simulink model "M2C_IM_CL_V1_NCADMM_Sim"  (R2023a)
settings: Solver=ode4  StartTime=0.0  StopTime=t_sim  FixedStep=tsim  RelTol=1e-3
model workspace (MAT data in the model file):
  global_can_baud_rate = '1000000'
  global_ip_addresses : object (value not decoded)
values from neighbouring files (symbols this model uses):
  A = [1 1 1 0 0 0 ... (first row only)    [M2C_init.m]    (also in MMCC_Sim_Script_BCD_activeset.m = -[1 0 0 1 0 0 1 0 0; 0 1 0 0 1 0 0 1 0; 0 0 1 0 0 1 0 0 1; -; MMCC_Sim_Script_BCD_activeset_LH.m = -[1 0 0 1 0 0 1 0 0; 0 1 0 0 1 0 0 1 0; 0 0 1 0 0 1 0 0 1; -)
  A11 = -(1/tau_sig)*eye(2)    [M2C_init.m]
  A21 = (Lm/tau_r)*eye(2)    [M2C_init.m]
  A_admm = zeros(2*Np, Np)    [M2C_init.m]
  A_cc = [1 0 ... (first row only)    [M2C_init.m]
  b_admm_1 = imax_admm*ones(2*Np,1)    [M2C_init.m]
  b_cc = Vmax_cc*ones(4,1)    [M2C_init.m]
  c_admm = -imax_admm*ones(Np,1)    [M2C_init.m]
  C_obs = [eye(2) zeros(2)]    [M2C_init.m]
  C_sm = 987e-6    (= 0.000987)    [M2C_init.m]
  G_cc = [1 1 ... (first row only)    [M2C_init.m]
  J_imag = [0 -1 ... (first row only)    [M2C_init.m]
  K_obsm = K_obs2'    [M2C_init.m]
  K_obsp = K_obs1'    [M2C_init.m]
  kr = Lm/Lr    (= 0.989061842659)    [M2C_init.m]
  L = 5e-3    (= 0.005)    [M2C_init.m]    (also in MMCC_Sim_Script_BCD_activeset.m = 0.02; MMCC_Sim_Script_BCD_activeset_LH.m = 0.02)
  Lsigmar = 2.6e-3    (= 0.0026)    [M2C_init.m]
  Lsigmas = 2.6e-3    (= 0.0026)    [M2C_init.m]
  N = [1/sqrt(3) 0;-1/(2*sqrt(3)) 1/2;-1/(2*sqrt(3)) -1/2;-1/sqrt(3) 0;1/(2*sqrt(3)) -1/2;1/(2*sqrt(3)) 1/2]    [M2C_init.m]    (also in MMCC_Sim_Script_BCD_activeset.m = null(A,'rational'); MMCC_Sim_Script_BCD_activeset_LH.m = [-0.4430   -0.4780    0.0994    0.0994)
  n = 4    [M2C_init.m]
  p = 2    [M2C_init.m]
  phirN = 1*Vb/ws_nom    [M2C_init.m]
  prmt_ADMM = [n, lambda_z, rho, lambda_e, C_sm, Np, imax_admm]    [M2C_init.m]
  prmt_bkpsi = [ts, Np, lambda_o, imax_admm]    [M2C_init.m]
  prmt_CCMPC = [ts, L, lambda_u, lambda_i, R, e]    [M2C_init.m]
  prmt_OBS = [ts, kr, sigma, Ls, tau_r]    [M2C_init.m]
  R = 0.2    [M2C_init.m]    (also in MMCC_Sim_Script_BCD_activeset.m = 0.001; MMCC_Sim_Script_BCD_activeset_LH.m = 0.001)
  Rr = 1.8    [M2C_init.m]
  Rs = 1.8    [M2C_init.m]
  Rsig = Rs + Rr*kr^2    (= 3.56083799149)    [M2C_init.m]
  SN = PN/FPn    (= 3703.7037037)    [M2C_init.m]
  T = [An ... (first row only)    [M2C_init.m]    (also in MMCC_Sim_Script_BCD_activeset.m = [1   0 ; -1/2  sqrt(3)/2; -1/2  -sqrt(3)/2]; MMCC_Sim_Script_BCD_activeset_LH.m = [1   0 ; -1/2  sqrt(3)/2; -1/2  -sqrt(3)/2])
  t_arranque = t_flux + 5/(dam*wn_flux) + 0.4    [M2C_init.m]
  t_flux = t_maq + 0.1    (= 0.3)    [M2C_init.m]
  t_load = t_arranque    [M2C_init.m]
  Tab0 = (1/3)*[2 -1 -1 ... (first row only)    [M2C_init.m]
  Tabc = [1 0; -.5 sqrt(3)/2; -.5 -sqrt(3)/2]    [M2C_init.m]
  tau_r = Lr/Rr    (= 0.132055555556)    [M2C_init.m]
  TN = PN/(nN*pi/30)    (= 19.7571653493)    [M2C_init.m]
  ts = 1/fs    (= 0.000166666666667)    [M2C_init.m]
  tsim = ts/40    (= 4.16666666667e-06)    [M2C_init.m]
  Vc0 = n*Vc_sm    (= 520)    [M2C_init.m]    (also in MMCC_Sim_Script_BCD_activeset.m = 18000; MMCC_Sim_Script_BCD_activeset_LH.m = 18000)
  Vc_sm = 130    [M2C_init.m]
  Vdc = n*Vc_sm    (= 520)    [M2C_init.m]
undefined symbols (not defined in the file or in its folder): Down, M2C_ADMM_Init_IM_V1, plecs, Up
libraries: spsIGBTDiodeLib x48, spsVoltageMeasurementLib x36, spsSeriesRLCBranchLib x30, spsCurrentMeasurementLib x10, eePwmGenerator x6, rtlab x3, dspstat3 x2, spsControlledVoltageSourceLib x2, spsDCVoltageSourceLib x2, opal_lib x1, dspfdesign x1, spsMeanLib x1
(part 4 of 6)

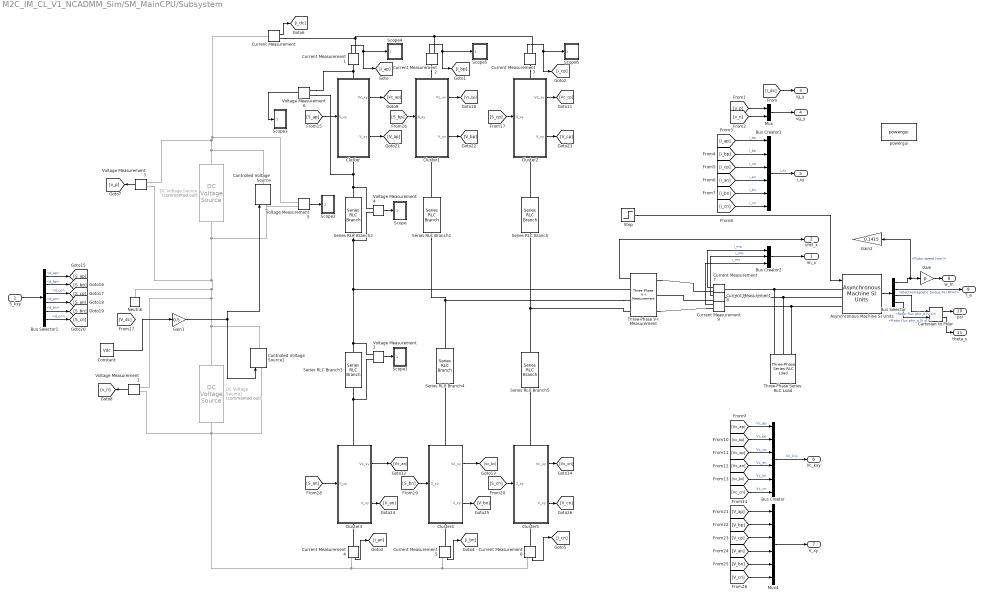
== system M2C_IM_CL_V1_NCADMM_Sim/SM_MainCPU/Subsystem ==
  S_kxy : Inport
  Asynchronous Machine SI Units : spsAsynchronousMachineSIUnitsLib/Asynchronous Machine SI Units  RotorType=Squirrel-cage  PresetModel=No  MechanicalLoad=Torque Tm  ShowDetailedParameters=on  ReferenceFrame=Rotor  Units=SI  MeasurementBus=off  NominalParameters=[3000 400 50]  VoltageRatio=1  Stator=[Rs Lsigmas]  Rotor=[Rr Lsigmar]  Cage1=[0.4155 0.002066]  Cage2=[0.4168 0.0003495]  Lm=Lm  Mechanical=[0.006 0.0057*0 p]  PolePairs=2  InitialConditions=[1 90 0 0 0 0 0 0]  SimulateSaturation=off  Saturation=[14.03593122, 27.81365428, 53.79336849, 72.68890987, 97.98006896, 148.6815601, 215.7428561, 302.9841135, 428.7778367 ; 230, 322, 414, 460, 506, 552, 598, 644, 690]  LoadFlowParameters=1492000  TsPowergui=0  TsBlock=tsim  IterativeModel=Trapezoidal non iterative  IterativeDiscreteModel=Trapezoidal non iterative  Pmec=0
  Bus Creator : BusCreator  Inputs=6
  Bus Creator1 : BusCreator  Inputs=6
  Bus Creator2 : BusCreator  Inputs=3
  Bus Selector : BusSelector  OutputSignals=Mechanical.Rotor speed (wm),Mechanical.Electromagnetic torque Te (N*m),Rotor measurements.Rotor flux phir_d (V s),Rotor measurements.Rotor flux phir_q (V s)
  Bus Selector1 : BusSelector  OutputSignals=S_p.d_ap,S_p.d_bp,S_p.d_cp,S_n.d_an,S_n.d_bn,S_n.d_cn
  Cartesian to Polar : simulink_extras/Transformations/Cartesian to Polar
  Cluster : Subsystem
      settings: PortSchema="{\"entries\":[{\"content\":{\"sides\":[{\"content\":{\"connectorIds\":[\"In1\"]},\"type\":\"ConnectorPlacement.EquallySpacedRectSide\",\"uuid\":\"19b6a211-5636-4e1a-b566-92ce17a08f23\"},{\"content\":{\"connectorIds\":[\"Out1\",\"Out2\"],\"side\":\"RIGHT\"},\"type\":\"ConnectorPlacement.EquallySpacedRectSide\",\"uuid\":\"483b1e0d-23ae-4dba-a621-2706d89ef2c0\"},{\"content\":{\"connectorIds\":[\"LConn1\"],\"side\":\"TOP\"},\"type\":\"ConnectorPlacement.EquallySpacedRectSide\",\"uuid\":\"4d4f4f94-f98d-4d38-ba04-9db58fc318a2\"},{\"content\":{\"connectorIds\":[\"RConn1\"],\"side\":\"BOTTOM\"},\"type\":\"ConnectorPlacement.EquallySpacedRectSide\",\"uuid\":\"4e2c39e0-8a4f-4729-a37c-1f4684d26f15\"}]},\"type\":\"ConnectorPlacement.EquallySpacedConnector\",\"uuid\":\"4c9a22d5-cdf0-40e5-b6bd-94d006c5c37f\"}],\"packageUris\":[\"http://schema.mathworks.com/mf0/Connector/R2020b\"],\"version\":\"1.0\"}"
  Cluster1 : Subsystem
      settings: PortSchema="{\"entries\":[{\"content\":{\"sides\":[{\"content\":{\"connectorIds\":[\"In1\"]},\"type\":\"ConnectorPlacement.EquallySpacedRectSide\",\"uuid\":\"19b6a211-5636-4e1a-b566-92ce17a08f23\"},{\"content\":{\"connectorIds\":[\"Out1\",\"Out2\"],\"side\":\"RIGHT\"},\"type\":\"ConnectorPlacement.EquallySpacedRectSide\",\"uuid\":\"483b1e0d-23ae-4dba-a621-2706d89ef2c0\"},{\"content\":{\"connectorIds\":[\"LConn1\"],\"side\":\"TOP\"},\"type\":\"ConnectorPlacement.EquallySpacedRectSide\",\"uuid\":\"4d4f4f94-f98d-4d38-ba04-9db58fc318a2\"},{\"content\":{\"connectorIds\":[\"RConn1\"],\"side\":\"BOTTOM\"},\"type\":\"ConnectorPlacement.EquallySpacedRectSide\",\"uuid\":\"4e2c39e0-8a4f-4729-a37c-1f4684d26f15\"}]},\"type\":\"ConnectorPlacement.EquallySpacedConnector\",\"uuid\":\"4c9a22d5-cdf0-40e5-b6bd-94d006c5c37f\"}],\"packageUris\":[\"http://schema.mathworks.com/mf0/Connector/R2020b\"],\"version\":\"1.0\"}"
  Cluster2 : Subsystem
      settings: PortSchema="{\"entries\":[{\"content\":{\"sides\":[{\"content\":{\"connectorIds\":[\"In1\"]},\"type\":\"ConnectorPlacement.EquallySpacedRectSide\",\"uuid\":\"19b6a211-5636-4e1a-b566-92ce17a08f23\"},{\"content\":{\"connectorIds\":[\"Out1\",\"Out2\"],\"side\":\"RIGHT\"},\"type\":\"ConnectorPlacement.EquallySpacedRectSide\",\"uuid\":\"483b1e0d-23ae-4dba-a621-2706d89ef2c0\"},{\"content\":{\"connectorIds\":[\"LConn1\"],\"side\":\"TOP\"},\"type\":\"ConnectorPlacement.EquallySpacedRectSide\",\"uuid\":\"4d4f4f94-f98d-4d38-ba04-9db58fc318a2\"},{\"content\":{\"connectorIds\":[\"RConn1\"],\"side\":\"BOTTOM\"},\"type\":\"ConnectorPlacement.EquallySpacedRectSide\",\"uuid\":\"4e2c39e0-8a4f-4729-a37c-1f4684d26f15\"}]},\"type\":\"ConnectorPlacement.EquallySpacedConnector\",\"uuid\":\"4c9a22d5-cdf0-40e5-b6bd-94d006c5c37f\"}],\"packageUris\":[\"http://schema.mathworks.com/mf0/Connector/R2020b\"],\"version\":\"1.0\"}"
  Cluster3 : Subsystem
      settings: PortSchema="{\"entries\":[{\"content\":{\"sides\":[{\"content\":{\"connectorIds\":[\"In1\"]},\"type\":\"ConnectorPlacement.EquallySpacedRectSide\",\"uuid\":\"19b6a211-5636-4e1a-b566-92ce17a08f23\"},{\"content\":{\"connectorIds\":[\"Out1\",\"Out2\"],\"side\":\"RIGHT\"},\"type\":\"ConnectorPlacement.EquallySpacedRectSide\",\"uuid\":\"483b1e0d-23ae-4dba-a621-2706d89ef2c0\"},{\"content\":{\"connectorIds\":[\"LConn1\"],\"side\":\"TOP\"},\"type\":\"ConnectorPlacement.EquallySpacedRectSide\",\"uuid\":\"4d4f4f94-f98d-4d38-ba04-9db58fc318a2\"},{\"content\":{\"connectorIds\":[\"RConn1\"],\"side\":\"BOTTOM\"},\"type\":\"ConnectorPlacement.EquallySpacedRectSide\",\"uuid\":\"4e2c39e0-8a4f-4729-a37c-1f4684d26f15\"}]},\"type\":\"ConnectorPlacement.EquallySpacedConnector\",\"uuid\":\"4c9a22d5-cdf0-40e5-b6bd-94d006c5c37f\"}],\"packageUris\":[\"http://schema.mathworks.com/mf0/Connector/R2020b\"],\"version\":\"1.0\"}"
  Cluster4 : Subsystem
      settings: PortSchema="{\"entries\":[{\"content\":{\"sides\":[{\"content\":{\"connectorIds\":[\"In1\"]},\"type\":\"ConnectorPlacement.EquallySpacedRectSide\",\"uuid\":\"19b6a211-5636-4e1a-b566-92ce17a08f23\"},{\"content\":{\"connectorIds\":[\"Out1\",\"Out2\"],\"side\":\"RIGHT\"},\"type\":\"ConnectorPlacement.EquallySpacedRectSide\",\"uuid\":\"483b1e0d-23ae-4dba-a621-2706d89ef2c0\"},{\"content\":{\"connectorIds\":[\"LConn1\"],\"side\":\"TOP\"},\"type\":\"ConnectorPlacement.EquallySpacedRectSide\",\"uuid\":\"4d4f4f94-f98d-4d38-ba04-9db58fc318a2\"},{\"content\":{\"connectorIds\":[\"RConn1\"],\"side\":\"BOTTOM\"},\"type\":\"ConnectorPlacement.EquallySpacedRectSide\",\"uuid\":\"4e2c39e0-8a4f-4729-a37c-1f4684d26f15\"}]},\"type\":\"ConnectorPlacement.EquallySpacedConnector\",\"uuid\":\"4c9a22d5-cdf0-40e5-b6bd-94d006c5c37f\"}],\"packageUris\":[\"http://schema.mathworks.com/mf0/Connector/R2020b\"],\"version\":\"1.0\"}"
  Cluster5 : Subsystem
      settings: PortSchema="{\"entries\":[{\"content\":{\"sides\":[{\"content\":{\"connectorIds\":[\"In1\"]},\"type\":\"ConnectorPlacement.EquallySpacedRectSide\",\"uuid\":\"19b6a211-5636-4e1a-b566-92ce17a08f23\"},{\"content\":{\"connectorIds\":[\"Out1\",\"Out2\"],\"side\":\"RIGHT\"},\"type\":\"ConnectorPlacement.EquallySpacedRectSide\",\"uuid\":\"483b1e0d-23ae-4dba-a621-2706d89ef2c0\"},{\"content\":{\"connectorIds\":[\"LConn1\"],\"side\":\"TOP\"},\"type\":\"ConnectorPlacement.EquallySpacedRectSide\",\"uuid\":\"4d4f4f94-f98d-4d38-ba04-9db58fc318a2\"},{\"content\":{\"connectorIds\":[\"RConn1\"],\"side\":\"BOTTOM\"},\"type\":\"ConnectorPlacement.EquallySpacedRectSide\",\"uuid\":\"4e2c39e0-8a4f-4729-a37c-1f4684d26f15\"}]},\"type\":\"ConnectorPlacement.EquallySpacedConnector\",\"uuid\":\"4c9a22d5-cdf0-40e5-b6bd-94d006c5c37f\"}],\"packageUris\":[\"http://schema.mathworks.com/mf0/Connector/R2020b\"],\"version\":\"1.0\"}"
  Constant : Constant  Value=Vdc  SampleTime=ts
  Controlled Voltage Source : spsControlledVoltageSourceLib/Controlled Voltage Source  Initialize=on  Source_Type=AC  Amplitude=0  Phase=0  Frequency=0  Measurements=None
  Controlled Voltage Source1 : spsControlledVoltageSourceLib/Controlled Voltage Source  Initialize=on  Source_Type=AC  Amplitude=0  Phase=0  Frequency=0  Measurements=None
  Current Measurement{,1..9} (10 alike) : spsCurrentMeasurementLib/Current Measurement  PhasorSimulation=off  OutputType=Complex  PSBequivalent=0
  DC Voltage Source : spsDCVoltageSourceLib/DC Voltage Source  Commented=on  Amplitude=Vdc/2  Measurements=None
  DC Voltage Source1 : spsDCVoltageSourceLib/DC Voltage Source  Commented=on  Amplitude=Vdc/2  Measurements=None
  Gain : Gain  Gain=p
  Gain1 : Gain  Gain=0.5
  Gain2 : Gain  Gain=0.1415
  Mux : Mux  Inputs=2
  Mux4 : Mux  Inputs=6
  Neutral : spsNeutralLib/Neutral  LConnTagsString=a  NodeNumber=10
      settings: AttributesFormatString=node %<NodeNumber>
  Scope : Subsystem  LoadFcn=plecs('sl', 300);  InitFcn=plecs('sl', 314);  StartFcn=plecs('sl', 308);  StopFcn=plecs('sl', 309);  mask{Settings=<binary blob, 1052 chars, not shown>}
      mask init:
      | plecs('sl', 315);
      settings: CopyFcn=plecs('sl', 303);  DeleteFcn=plecs('sl', 305);  UndoDeleteFcn=plecs('sl', 306);  PreSaveFcn=plecs('sl', 311);  NameChangeFcn=plecs('sl', 310);  DestroyFcn=plecs('sl', 307);  OpenFcn=plecs('sl', 302);  ErrorFcn=plerrorfcn
      mask Display: plot([0.1 0.9 0.9 0.1 0.1], [0.9 0.9 0.5 0.5 0.9])
  Scope1 : Subsystem  LoadFcn=plecs('sl', 300);  InitFcn=plecs('sl', 314);  StartFcn=plecs('sl', 308);  StopFcn=plecs('sl', 309);  mask{Settings=<binary blob, 1052 chars, not shown>}
      mask init:
      | plecs('sl', 315);
      settings: CopyFcn=plecs('sl', 303);  DeleteFcn=plecs('sl', 305);  UndoDeleteFcn=plecs('sl', 306);  PreSaveFcn=plecs('sl', 311);  NameChangeFcn=plecs('sl', 310);  DestroyFcn=plecs('sl', 307);  OpenFcn=plecs('sl', 302);  ErrorFcn=plerrorfcn
      mask Display: plot([0.1 0.9 0.9 0.1 0.1], [0.9 0.9 0.5 0.5 0.9])
  Scope2 : Subsystem  LoadFcn=plecs('sl', 300);  InitFcn=plecs('sl', 314);  StartFcn=plecs('sl', 308);  StopFcn=plecs('sl', 309);  mask{Settings=<binary blob, 1052 chars, not shown>}
      mask init:
      | plecs('sl', 315);
      settings: CopyFcn=plecs('sl', 303);  DeleteFcn=plecs('sl', 305);  UndoDeleteFcn=plecs('sl', 306);  PreSaveFcn=plecs('sl', 311);  NameChangeFcn=plecs('sl', 310);  DestroyFcn=plecs('sl', 307);  OpenFcn=plecs('sl', 302);  ErrorFcn=plerrorfcn
      mask Display: plot([0.1 0.9 0.9 0.1 0.1], [0.9 0.9 0.5 0.5 0.9])
  Scope3 : Subsystem  LoadFcn=plecs('sl', 300);  InitFcn=plecs('sl', 314);  StartFcn=plecs('sl', 308);  StopFcn=plecs('sl', 309);  mask{Settings=<binary blob, 1052 chars, not shown>}
      mask init:
      | plecs('sl', 315);
      settings: CopyFcn=plecs('sl', 303);  DeleteFcn=plecs('sl', 305);  UndoDeleteFcn=plecs('sl', 306);  PreSaveFcn=plecs('sl', 311);  NameChangeFcn=plecs('sl', 310);  DestroyFcn=plecs('sl', 307);  OpenFcn=plecs('sl', 302);  ErrorFcn=plerrorfcn
      mask Display: plot([0.1 0.9 0.9 0.1 0.1], [0.9 0.9 0.5 0.5 0.9])
  Scope4 : Subsystem  LoadFcn=plecs('sl', 300);  InitFcn=plecs('sl', 314);  StartFcn=plecs('sl', 308);  StopFcn=plecs('sl', 309);  mask{Settings=<binary blob, 236 chars, not shown>}
      mask init:
      | plecs('sl', 315);
      settings: CopyFcn=plecs('sl', 303);  DeleteFcn=plecs('sl', 305);  UndoDeleteFcn=plecs('sl', 306);  PreSaveFcn=plecs('sl', 311);  NameChangeFcn=plecs('sl', 310);  DestroyFcn=plecs('sl', 307);  OpenFcn=plecs('sl', 302);  ErrorFcn=plerrorfcn
      mask Display: plot([0.1 0.9 0.9 0.1 0.1], [0.9 0.9 0.5 0.5 0.9])
  Scope5 : Subsystem  LoadFcn=plecs('sl', 300);  InitFcn=plecs('sl', 314);  StartFcn=plecs('sl', 308);  StopFcn=plecs('sl', 309);  mask{Settings=<binary blob, 236 chars, not shown>}
      mask init:
      | plecs('sl', 315);
      settings: CopyFcn=plecs('sl', 303);  DeleteFcn=plecs('sl', 305);  UndoDeleteFcn=plecs('sl', 306);  PreSaveFcn=plecs('sl', 311);  NameChangeFcn=plecs('sl', 310);  DestroyFcn=plecs('sl', 307);  OpenFcn=plecs('sl', 302);  ErrorFcn=plerrorfcn
      mask Display: plot([0.1 0.9 0.9 0.1 0.1], [0.9 0.9 0.5 0.5 0.9])
  Scope6 : Subsystem  LoadFcn=plecs('sl', 300);  InitFcn=plecs('sl', 314);  StartFcn=plecs('sl', 308);  StopFcn=plecs('sl', 309);  mask{Settings=<binary blob, 236 chars, not shown>}
      mask init:
      | plecs('sl', 315);
      settings: CopyFcn=plecs('sl', 303);  DeleteFcn=plecs('sl', 305);  UndoDeleteFcn=plecs('sl', 306);  PreSaveFcn=plecs('sl', 311);  NameChangeFcn=plecs('sl', 310);  DestroyFcn=plecs('sl', 307);  OpenFcn=plecs('sl', 302);  ErrorFcn=plerrorfcn
      mask Display: plot([0.1 0.9 0.9 0.1 0.1], [0.9 0.9 0.5 0.5 0.9])
  Series RLC Branch{,1..5} (6 alike) : spsSeriesRLCBranchLib/Series RLC Branch  LConnTagsString=__new0  RConnTagsString=__new0  BranchType=RL  Resistance=R  Inductance=L  SetiL0=off  InitialCurrent=0  Capacitance=1e-6  Setx0=off  InitialVoltage=0  Measurements=None
  Step : Step  Time=t_load+2  After=TN*0.4  SampleTime=0
  Three-Phase Series RLC Load : spsThreePhaseSeriesRLCLoadLib/Three-Phase Series RLC Load  LConnTagsString=A|B|C  Configuration=Y (floating)  NominalVoltage=VLLN  Vabc=[1e3 1e3 1e3]  Vabcp=[1e3 1e3 1e3]  NominalFrequency=50  UnbalancedPower=off  ActivePower=SN*0.01  InductivePower=0  CapacitivePower=0  Pabc=[10e3 9e3 11e3]  QLabc=[100 90 110]  QCabc=[100 90 110]  Pabcp=[10e3 9e3 11e3]  QLabcp=[100 90 110]  QCabcp=[100 90 110]  Measurements=None  LoadType=constant Z
  Three-Phase V-I Measurement : spsThreePhaseVIMeasurementLib/Three-Phase V-I Measurement  VoltageMeasurement=phase-to-phase  SetLabelV=off  LabelV=Vabc  Vpu=off  VpuLL=off  CurrentMeasurement=no  SetLabelI=off  LabelI=Iabc  Ipu=off  Pbase=100e6  Vbase=500e3  OutputType=Complex  PhasorSimulation=off  PSBequivalent=0
  Voltage Measurement{1..6} (6 alike) : spsVoltageMeasurementLib/Voltage Measurement  PhasorSimulation=off  OutputType=Complex  PSBequivalent=0
  powergui : spspowerguiLib/powergui  Priority=1  SimulationMode=Discrete  SampleTime=tsim  frequency=60  Iterations=50  frequencyindice=0  Pbase=100e6  ErrMax=1e-4  UnitsV=kV  UnitsW=MW  buscounter=0  FunctionMessages=off  echomessages=off  EnableUseOfTLC=off  CurrentSourceSwitches=off  DisableSnubberDevices=off  DisableRonSwitches=off  DisableVfSwitches=off  DisplayEquations=off  AutomaticDiscreteSolvers=off  SolverType=Tustin/Backward Euler (TBE)  Interpol=off  ExternalGateDelay=off  methode=off  Ts=100  x0status=blocks  SPID=on  SwTol=0  HookPort=off  NonlinearTolerance=1e-4  nMaxIteration=100  ContinueOnMaxIteration=off  RestoreLinks=warning  ResistiveCurrentMeasurement=off  Frange=[0:2:500]  Ylog=off  Xlog=on  ShowGrid=off  save=off  variable=ZData  structure=0  ZoomFFT=off  StartTime=0.0  cycles=1  DisplayStyle=1  fundamental=60  FreqAxis=off  MaxFrequency=1000  frequencyindicesteady=1  RmsSteady=1  display=off
  im_x : Outport
  vmll_x : Outport  Port=2
  ig_y : Outport  Port=3
  vg_y : Outport  Port=4
  i_xy : Outport  Port=5
  Vc_kxy : Outport  Port=6
  V_xy : Outport  Port=7
  w_m : Outport  Port=8
  T_e : Outport  Port=9
  psi : Outport  Port=10
  theta_s : Outport  Port=11
  wires:
  Three-Phase V-I Measurement/1 -> vmll_x/1
  [i_dc] -> ig_y/1
  Voltage Measurement3/1 -> [v_p]
  Voltage Measurement1/1 -> [v_n]
  [v_p] -> Mux/1
  [v_n] -> Mux/2
  Mux/1 -> vg_y/1
  [i_ap] -> Bus Creator1/1  "i_ap"
  [i_bp] -> Bus Creator1/2  "i_bp"
  [i_cp] -> Bus Creator1/3  "i_cp"
  [i_an] -> Bus Creator1/4  "i_an"
  [i_bn] -> Bus Creator1/5  "i_bn"
  [i_cn] -> Bus Creator1/6  "i_cn"
  Bus Creator1/1 -> i_xy/1  "i_xy"
  Cluster/1(Vc_xy) -> [Vc_ap]
  Cluster1/1(Vc_xy) -> [Vc_bp]
  Cluster2/1(Vc_xy) -> [Vc_cp]
  Cluster3/1(Vc_xy) -> [Vc_an]
  Cluster4/1(Vc_xy) -> [Vc_bn]
  Cluster5/1(Vc_xy) -> [Vc_cn]
  [Vc_ap] -> Bus Creator/1  "Vc_ap"
  [Vc_bp] -> Bus Creator/2  "Vc_bp"
  [Vc_cp] -> Bus Creator/3  "Vc_cp"
  [Vc_an] -> Bus Creator/4  "Vc_an"
  [Vc_cn] -> Bus Creator/6  "Vc_cn"
  [Vc_bn] -> Bus Creator/5  "Vc_bn"
  Bus Creator/1 -> Vc_kxy/1  "Vc_kxy"
  Bus Selector1/6 -> [S_cn]  "<d_cn>"
  Bus Selector1/5 -> [S_bn]  "<d_bn>"
  Bus Selector1/4 -> [S_an]  "<d_an>"
  Bus Selector1/3 -> [S_cp]  "<d_cp>"
  Bus Selector1/2 -> [S_bp]  "<d_bp>"
  Bus Selector1/1 -> [S_ap]  "<d_ap>"
  [S_ap] -> Cluster/1(S_xy)
  [S_bp] -> Cluster1/1(S_xy)
  [S_cp] -> Cluster2/1(S_xy)
  [S_an] -> Cluster3/1(S_xy)
  [S_bn] -> Cluster4/1(S_xy)
  [S_cn] -> Cluster5/1(S_xy)
  Bus Creator2/1 -> im_x/1
  Current Measurement1/1 -> Scope4/1(1), [i_ap]
  Current Measurement2/1 -> Scope5/1(1), [i_bp]
  Current Measurement3/1 -> Scope6/1(1), [i_cp]
  Current Measurement4/1 -> [i_an]
  Current Measurement5/1 -> [i_bn]
  Current Measurement6/1 -> [i_cn]
  Current Measurement/1 -> [i_dc]
  Current Measurement7/1 -> Bus Creator2/1  "i_ma"
  Current Measurement8/1 -> Bus Creator2/2  "i_mb"
  Current Measurement9/1 -> Bus Creator2/3  "i_mc"
  Cluster/2(V_xy) -> [V_ap]
  Cluster1/2(V_xy) -> [V_bp]
  Cluster2/2(V_xy) -> [V_cp]
  Cluster4/2(V_xy) -> [V_bn]
  Cluster5/2(V_xy) -> [V_cn]
  Cluster3/2(V_xy) -> [V_an]
  Mux4/1 -> V_xy/1
  [V_ap] -> Mux4/1
  [V_bp] -> Mux4/2
  [V_cp] -> Mux4/3
  [V_an] -> Mux4/4
  [V_bn] -> Mux4/5
  [V_cn] -> Mux4/6
  S_kxy/1 -> Bus Selector1/1
  Constant/1 -> Gain1/1
  Gain1/1 -> Controlled Voltage Source/1, Controlled Voltage Source1/1
  Asynchronous Machine SI Units/1 -> Bus Selector/1
  Bus Selector/1 -> Gain2/1, Gain/1  "<Rotor speed (wm)>"
  Gain/1 -> w_m/1
  Bus Selector/2 -> T_e/1  "<Electromagnetic torque Te (N*m)>"
  Cartesian to Polar/1 -> psi/1
  Cartesian to Polar/2 -> theta_s/1
  Bus Selector/3 -> Cartesian to Polar/1  "<Rotor flux phir_d (V s)>"
  Bus Selector/4 -> Cartesian to Polar/2  "<Rotor flux phir_q (V s)>"
  Step/1 -> Asynchronous Machine SI Units/1
  Voltage Measurement4/1 -> Scope/1(1)
  Voltage Measurement2/1 -> Scope1/1(1)
  Voltage Measurement5/1 -> Scope2/1(1)
  Voltage Measurement6/1 -> Scope3/1(1)
  connections:
  Series RLC Branch/LConn1 -- Cluster2/RConn1
  Series RLC Branch1/LConn1 -- Cluster1/RConn1
  Cluster/RConn1 -- Voltage Measurement6/LConn2 -- Voltage Measurement4/LConn1 -- Series RLC Branch2/LConn1
  Current Measurement1/RConn1 -- Current Measurement/RConn1 -- Current Measurement3/RConn1 -- Current Measurement2/RConn1
  DC Voltage Source1/LConn1 -- Controlled Voltage Source1/LConn1 -- Current Measurement4/RConn1 -- Current Measurement6/RConn1 -- Current Measurement5/RConn1 -- Voltage Measurement1/LConn1
  DC Voltage Source/RConn1 -- Controlled Voltage Source/RConn1 -- Voltage Measurement5/LConn1 -- Current Measurement/LConn1 -- Voltage Measurement3/LConn1
  Series RLC Branch3/LConn1 -- Voltage Measurement2/LConn1 -- Cluster3/LConn1
  Series RLC Branch4/LConn1 -- Cluster4/LConn1
  Series RLC Branch5/LConn1 -- Cluster5/LConn1
  Current Measurement1/LConn1 -- Voltage Measurement6/LConn1 -- Cluster/LConn1
  Current Measurement2/LConn1 -- Cluster1/LConn1
  Current Measurement3/LConn1 -- Cluster2/LConn1
  Current Measurement4/LConn1 -- Cluster3/RConn1
  Current Measurement5/LConn1 -- Cluster4/RConn1
  Current Measurement6/LConn1 -- Cluster5/RConn1
  Current Measurement7/RConn1 -- Three-Phase V-I Measurement/LConn1
  Current Measurement8/RConn1 -- Three-Phase V-I Measurement/LConn2
  Current Measurement9/RConn1 -- Three-Phase V-I Measurement/LConn3
  Three-Phase Series RLC Load/LConn1 -- Asynchronous Machine SI Units/LConn1 -- Current Measurement7/LConn1
  Three-Phase V-I Measurement/RConn3 -- Series RLC Branch/RConn1 -- Series RLC Branch5/RConn1
  DC Voltage Source/LConn1 -- Voltage Measurement5/LConn2 -- Controlled Voltage Source/LConn1 -- Neutral/LConn1 -- Voltage Measurement1/LConn2 -- Controlled Voltage Source1/RConn1 -- DC Voltage Source1/RConn1 -- Voltage Measurement3/LConn2
  Three-Phase V-I Measurement/RConn2 -- Series RLC Branch1/RConn1 -- Series RLC Branch4/RConn1
  Three-Phase Series RLC Load/LConn2 -- Asynchronous Machine SI Units/LConn2 -- Current Measurement8/LConn1
  Three-Phase Series RLC Load/LConn3 -- Asynchronous Machine SI Units/LConn3 -- Current Measurement9/LConn1
  Voltage Measurement4/LConn2 -- Three-Phase V-I Measurement/RConn1 -- Voltage Measurement2/LConn2 -- Series RLC Branch3/RConn1 -- Series RLC Branch2/RConn1

== system M2C_IM_CL_V1_NCADMM_Sim/SM_MainCPU/V REFS1 ==
  1 : Inport
  2 : Inport  Port=2
  3 : Inport  Port=3
  " 1 " : DataTypeConversion
  " 2 " : DataTypeConversion
  " 3 " : DataTypeConversion
  " InputMux " : Mux  Inputs=3
  " S-Function " : S-Function  FunctionName=plecs  SFunctionDeploymentMode=off  EnableBusSupport=off
  wires:
  " InputMux "/1 -> " S-Function "/1
  1/1 -> " 1 "/1
  " 1 "/1 -> " InputMux "/1
  2/1 -> " 2 "/1
  " 2 "/1 -> " InputMux "/2
  3/1 -> " 3 "/1
  " 3 "/1 -> " InputMux "/3

== system M2C_IM_CL_V1_NCADMM_Sim/SM_MainCPU/LCB1/Scope ==
  1 : Inport
  " InputMux " : Subsystem
      mask Display: disp('Mux')
  " S-Function " : S-Function  FunctionName=plecs  SFunctionDeploymentMode=off  EnableBusSupport=off
  wires:
  1/1 -> " InputMux "/1(In1)
  " InputMux "/1(Out) -> " S-Function "/1

== system M2C_IM_CL_V1_NCADMM_Sim/SM_MainCPU/LCB1/Scope1 ==
  1 : Inport
  " InputMux " : Subsystem
      mask Display: disp('Mux')
  " S-Function " : S-Function  FunctionName=plecs  SFunctionDeploymentMode=off  EnableBusSupport=off
  wires:
  1/1 -> " InputMux "/1(In1)
  " InputMux "/1(Out) -> " S-Function "/1

== system M2C_IM_CL_V1_NCADMM_Sim/SM_MainCPU/LCB1/Scope2 ==
  1 : Inport
  " InputMux " : Subsystem
      mask Display: disp('Mux')
  " S-Function " : S-Function  FunctionName=plecs  SFunctionDeploymentMode=off  EnableBusSupport=off
  wires:
  1/1 -> " InputMux "/1(In1)
  " InputMux "/1(Out) -> " S-Function "/1

== system M2C_IM_CL_V1_NCADMM_Sim/SM_MainCPU/LCB1/Scope5 ==
  1 : Inport
  " InputMux " : Subsystem
      mask Display: disp('Mux')
  " S-Function " : S-Function  FunctionName=plecs  SFunctionDeploymentMode=off  EnableBusSupport=off
  wires:
  1/1 -> " InputMux "/1(In1)
  " InputMux "/1(Out) -> " S-Function "/1

== system M2C_IM_CL_V1_NCADMM_Sim/SM_MainCPU/Scope/ InputMux  ==
  In1 : Inport
  Convert1 : DataTypeConversion
  Mux : Mux  Inputs=1
  Out : Outport
  wires:
  Convert1/1 -> Mux/1
  In1/1 -> Convert1/1
  Mux/1 -> Out/1

== system M2C_IM_CL_V1_NCADMM_Sim/SM_MainCPU/Scope1/ InputMux  ==
  In1 : Inport
  Convert1 : DataTypeConversion
  Mux : Mux  Inputs=1
  Out : Outport
  wires:
  Convert1/1 -> Mux/1
  In1/1 -> Convert1/1
  Mux/1 -> Out/1

== system M2C_IM_CL_V1_NCADMM_Sim/SM_MainCPU/Scope10/ InputMux  ==
  In1 : Inport
  Convert1 : DataTypeConversion
  Mux : Mux  Inputs=1
  Out : Outport
  wires:
  Convert1/1 -> Mux/1
  In1/1 -> Convert1/1
  Mux/1 -> Out/1

== system M2C_IM_CL_V1_NCADMM_Sim/SM_MainCPU/Scope11/ InputMux  ==
  In1 : Inport
  Convert1 : DataTypeConversion
  Mux : Mux  Inputs=1
  Out : Outport
  wires:
  Convert1/1 -> Mux/1
  In1/1 -> Convert1/1
  Mux/1 -> Out/1

== system M2C_IM_CL_V1_NCADMM_Sim/SM_MainCPU/Scope12/ InputMux  ==
  In1 : Inport
  Convert1 : DataTypeConversion
  Mux : Mux  Inputs=1
  Out : Outport
  wires:
  Convert1/1 -> Mux/1
  In1/1 -> Convert1/1
  Mux/1 -> Out/1

== system M2C_IM_CL_V1_NCADMM_Sim/SM_MainCPU/Scope13/ InputMux  ==
  In1 : Inport
  Convert1 : DataTypeConversion
  Mux : Mux  Inputs=1
  Out : Outport
  wires:
  Convert1/1 -> Mux/1
  In1/1 -> Convert1/1
  Mux/1 -> Out/1

== system M2C_IM_CL_V1_NCADMM_Sim/SM_MainCPU/Scope14/ InputMux  ==
  In1 : Inport
  Convert1 : DataTypeConversion
  Mux : Mux  Inputs=1
  Out : Outport
  wires:
  Convert1/1 -> Mux/1
  In1/1 -> Convert1/1
  Mux/1 -> Out/1

== system M2C_IM_CL_V1_NCADMM_Sim/SM_MainCPU/Scope15/ InputMux  ==
  In1 : Inport
  Convert1 : DataTypeConversion
  Mux : Mux  Inputs=1
  Out : Outport
  wires:
  Convert1/1 -> Mux/1
  In1/1 -> Convert1/1
  Mux/1 -> Out/1

== system M2C_IM_CL_V1_NCADMM_Sim/SM_MainCPU/Scope16/ InputMux  ==
  In1 : Inport
  Convert1 : DataTypeConversion
  Mux : Mux  Inputs=1
  Out : Outport
  wires:
  Convert1/1 -> Mux/1
  In1/1 -> Convert1/1
  Mux/1 -> Out/1

== system M2C_IM_CL_V1_NCADMM_Sim/SM_MainCPU/Scope17/ InputMux  ==
  In1 : Inport
  Convert1 : DataTypeConversion
  Mux : Mux  Inputs=1
  Out : Outport
  wires:
  Convert1/1 -> Mux/1
  In1/1 -> Convert1/1
  Mux/1 -> Out/1

== system M2C_IM_CL_V1_NCADMM_Sim/SM_MainCPU/Scope18/ InputMux  ==
  In1 : Inport
  Convert1 : DataTypeConversion
  Mux : Mux  Inputs=1
  Out : Outport
  wires:
  Convert1/1 -> Mux/1
  In1/1 -> Convert1/1
  Mux/1 -> Out/1

== system M2C_IM_CL_V1_NCADMM_Sim/SM_MainCPU/Scope19/ InputMux  ==
  In1 : Inport
  Convert1 : DataTypeConversion
  Mux : Mux  Inputs=1
  Out : Outport
  wires:
  Convert1/1 -> Mux/1
  In1/1 -> Convert1/1
  Mux/1 -> Out/1

== system M2C_IM_CL_V1_NCADMM_Sim/SM_MainCPU/Scope2/ InputMux  ==
  In1 : Inport
  Convert1 : DataTypeConversion
  Mux : Mux  Inputs=1
  Out : Outport
  wires:
  Convert1/1 -> Mux/1
  In1/1 -> Convert1/1
  Mux/1 -> Out/1

== system M2C_IM_CL_V1_NCADMM_Sim/SM_MainCPU/Scope20/ InputMux  ==
  In1 : Inport
  Convert1 : DataTypeConversion
  Mux : Mux  Inputs=1
  Out : Outport
  wires:
  Convert1/1 -> Mux/1
  In1/1 -> Convert1/1
  Mux/1 -> Out/1

== system M2C_IM_CL_V1_NCADMM_Sim/SM_MainCPU/Scope21/ InputMux  ==
  In1 : Inport
  Convert1 : DataTypeConversion
  Mux : Mux  Inputs=1
  Out : Outport
  wires:
  Convert1/1 -> Mux/1
  In1/1 -> Convert1/1
  Mux/1 -> Out/1

== system M2C_IM_CL_V1_NCADMM_Sim/SM_MainCPU/Scope22/ InputMux  ==
  In1 : Inport
  Convert1 : DataTypeConversion
  Mux : Mux  Inputs=1
  Out : Outport
  wires:
  Convert1/1 -> Mux/1
  In1/1 -> Convert1/1
  Mux/1 -> Out/1

== system M2C_IM_CL_V1_NCADMM_Sim/SM_MainCPU/Scope24/ InputMux  ==
  In1 : Inport
  Convert1 : DataTypeConversion
  Mux : Mux  Inputs=1
  Out : Outport
  wires:
  Convert1/1 -> Mux/1
  In1/1 -> Convert1/1
  Mux/1 -> Out/1

== system M2C_IM_CL_V1_NCADMM_Sim/SM_MainCPU/Scope25/ InputMux  ==
  In1 : Inport
  Convert1 : DataTypeConversion
  Mux : Mux  Inputs=1
  Out : Outport
  wires:
  Convert1/1 -> Mux/1
  In1/1 -> Convert1/1
  Mux/1 -> Out/1

== system M2C_IM_CL_V1_NCADMM_Sim/SM_MainCPU/Scope26/ InputMux  ==
  In1 : Inport
  Convert1 : DataTypeConversion
  Mux : Mux  Inputs=1
  Out : Outport
  wires:
  Convert1/1 -> Mux/1
  In1/1 -> Convert1/1
  Mux/1 -> Out/1

== system M2C_IM_CL_V1_NCADMM_Sim/SM_MainCPU/Scope27/ InputMux  ==
  In1 : Inport
  Convert1 : DataTypeConversion
  Mux : Mux  Inputs=1
  Out : Outport
  wires:
  Convert1/1 -> Mux/1
  In1/1 -> Convert1/1
  Mux/1 -> Out/1

== system M2C_IM_CL_V1_NCADMM_Sim/SM_MainCPU/Scope28/ InputMux  ==
  In1 : Inport
  Convert1 : DataTypeConversion
  Mux : Mux  Inputs=1
  Out : Outport
  wires:
  Convert1/1 -> Mux/1
  In1/1 -> Convert1/1
  Mux/1 -> Out/1

== system M2C_IM_CL_V1_NCADMM_Sim/SM_MainCPU/Scope29/ InputMux  ==
  In1 : Inport
  Convert1 : DataTypeConversion
  Mux : Mux  Inputs=1
  Out : Outport
  wires:
  Convert1/1 -> Mux/1
  In1/1 -> Convert1/1
  Mux/1 -> Out/1

== system M2C_IM_CL_V1_NCADMM_Sim/SM_MainCPU/Scope3/ InputMux  ==
  In1 : Inport
  Convert1 : DataTypeConversion
  Mux : Mux  Inputs=1
  Out : Outport
  wires:
  Convert1/1 -> Mux/1
  In1/1 -> Convert1/1
  Mux/1 -> Out/1

== system M2C_IM_CL_V1_NCADMM_Sim/SM_MainCPU/Scope30/ InputMux  ==
  In1 : Inport
  Convert1 : DataTypeConversion
  Mux : Mux  Inputs=1
  Out : Outport
  wires:
  Convert1/1 -> Mux/1
  In1/1 -> Convert1/1
  Mux/1 -> Out/1

== system M2C_IM_CL_V1_NCADMM_Sim/SM_MainCPU/Scope31/ InputMux  ==
  In1 : Inport
  Convert1 : DataTypeConversion
  Mux : Mux  Inputs=1
  Out : Outport
  wires:
  Convert1/1 -> Mux/1
  In1/1 -> Convert1/1
  Mux/1 -> Out/1

== system M2C_IM_CL_V1_NCADMM_Sim/SM_MainCPU/Scope33/ InputMux  ==
  In1 : Inport
  Convert1 : DataTypeConversion
  Mux : Mux  Inputs=1
  Out : Outport
  wires:
  Convert1/1 -> Mux/1
  In1/1 -> Convert1/1
  Mux/1 -> Out/1

== system M2C_IM_CL_V1_NCADMM_Sim/SM_MainCPU/Scope34/ InputMux  ==
  In1 : Inport
  Convert1 : DataTypeConversion
  Mux : Mux  Inputs=1
  Out : Outport
  wires:
  Convert1/1 -> Mux/1
  In1/1 -> Convert1/1
  Mux/1 -> Out/1

== system M2C_IM_CL_V1_NCADMM_Sim/SM_MainCPU/Scope35/ InputMux  ==
  In1 : Inport
  Convert1 : DataTypeConversion
  Mux : Mux  Inputs=1
  Out : Outport
  wires:
  Convert1/1 -> Mux/1
  In1/1 -> Convert1/1
  Mux/1 -> Out/1

== system M2C_IM_CL_V1_NCADMM_Sim/SM_MainCPU/Scope36/ InputMux  ==
  In1 : Inport
  Convert1 : DataTypeConversion
  Mux : Mux  Inputs=1
  Out : Outport
  wires:
  Convert1/1 -> Mux/1
  In1/1 -> Convert1/1
  Mux/1 -> Out/1

== system M2C_IM_CL_V1_NCADMM_Sim/SM_MainCPU/Scope37/ InputMux  ==
  In1 : Inport
  Convert1 : DataTypeConversion
  Mux : Mux  Inputs=1
  Out : Outport
  wires:
  Convert1/1 -> Mux/1
  In1/1 -> Convert1/1
  Mux/1 -> Out/1

== system M2C_IM_CL_V1_NCADMM_Sim/SM_MainCPU/Scope38/ InputMux  ==
  In1 : Inport
  Convert1 : DataTypeConversion
  Mux : Mux  Inputs=1
  Out : Outport
  wires:
  Convert1/1 -> Mux/1
  In1/1 -> Convert1/1
  Mux/1 -> Out/1

== system M2C_IM_CL_V1_NCADMM_Sim/SM_MainCPU/Scope39/ InputMux  ==
  In1 : Inport
  Convert1 : DataTypeConversion
  Mux : Mux  Inputs=1
  Out : Outport
  wires:
  Convert1/1 -> Mux/1
  In1/1 -> Convert1/1
  Mux/1 -> Out/1

== system M2C_IM_CL_V1_NCADMM_Sim/SM_MainCPU/Scope4/ InputMux  ==
  In1 : Inport
  Convert1 : DataTypeConversion
  Mux : Mux  Inputs=1
  Out : Outport
  wires:
  Convert1/1 -> Mux/1
  In1/1 -> Convert1/1
  Mux/1 -> Out/1

== system M2C_IM_CL_V1_NCADMM_Sim/SM_MainCPU/Scope40/ InputMux  ==
  In1 : Inport
  Convert1 : DataTypeConversion
  Mux : Mux  Inputs=1
  Out : Outport
  wires:
  Convert1/1 -> Mux/1
  In1/1 -> Convert1/1
  Mux/1 -> Out/1

== system M2C_IM_CL_V1_NCADMM_Sim/SM_MainCPU/Scope41/ InputMux  ==
  In1 : Inport
  Convert1 : DataTypeConversion
  Mux : Mux  Inputs=1
  Out : Outport
  wires:
  Convert1/1 -> Mux/1
  In1/1 -> Convert1/1
  Mux/1 -> Out/1

== system M2C_IM_CL_V1_NCADMM_Sim/SM_MainCPU/Scope42/ InputMux  ==
  In1 : Inport
  Convert1 : DataTypeConversion
  Mux : Mux  Inputs=1
  Out : Outport
  wires:
  Convert1/1 -> Mux/1
  In1/1 -> Convert1/1
  Mux/1 -> Out/1

== system M2C_IM_CL_V1_NCADMM_Sim/SM_MainCPU/Scope5/ InputMux  ==
  In1 : Inport
  Convert1 : DataTypeConversion
  Mux : Mux  Inputs=1
  Out : Outport
  wires:
  Convert1/1 -> Mux/1
  In1/1 -> Convert1/1
  Mux/1 -> Out/1

== system M2C_IM_CL_V1_NCADMM_Sim/SM_MainCPU/Scope6/ InputMux  ==
  In1 : Inport
  Convert1 : DataTypeConversion
  Mux : Mux  Inputs=1
  Out : Outport
  wires:
  Convert1/1 -> Mux/1
  In1/1 -> Convert1/1
  Mux/1 -> Out/1

== system M2C_IM_CL_V1_NCADMM_Sim/SM_MainCPU/Scope7/ InputMux  ==
  In1 : Inport
  Convert1 : DataTypeConversion
  Mux : Mux  Inputs=1
  Out : Outport
  wires:
  Convert1/1 -> Mux/1
  In1/1 -> Convert1/1
  Mux/1 -> Out/1

== system M2C_IM_CL_V1_NCADMM_Sim/SM_MainCPU/Scope8/ InputMux  ==
  In1 : Inport
  Convert1 : DataTypeConversion
  Mux : Mux  Inputs=1
  Out : Outport
  wires:
  Convert1/1 -> Mux/1
  In1/1 -> Convert1/1
  Mux/1 -> Out/1

== system M2C_IM_CL_V1_NCADMM_Sim/SM_MainCPU/Scope9/ InputMux  ==
  In1 : Inport
  Convert1 : DataTypeConversion
  Mux : Mux  Inputs=1
  Out : Outport
  wires:
  Convert1/1 -> Mux/1
  In1/1 -> Convert1/1
  Mux/1 -> Out/1

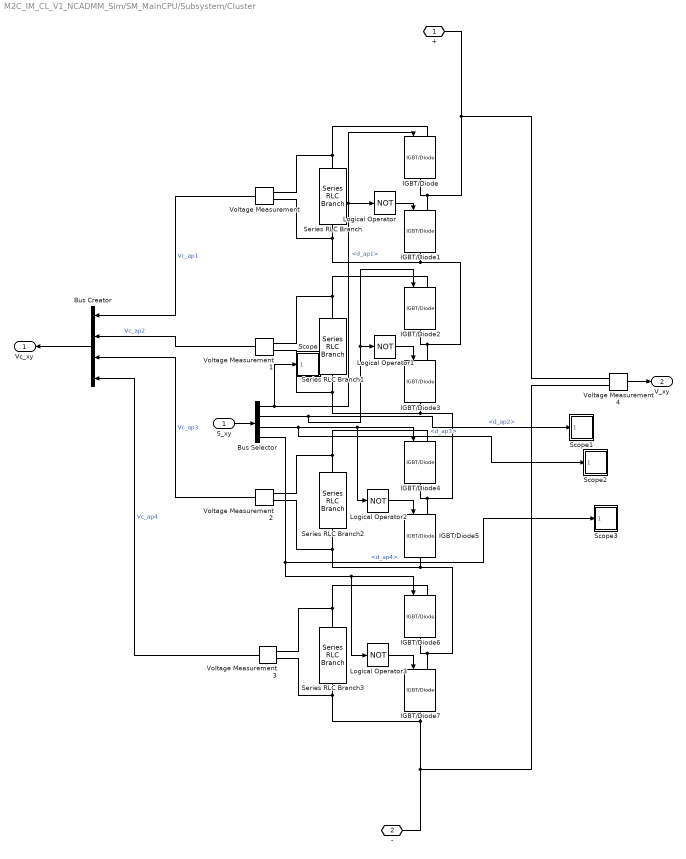
== system M2C_IM_CL_V1_NCADMM_Sim/SM_MainCPU/Subsystem/Cluster ==
  S_xy : Inport
  Bus Creator : BusCreator  Inputs=4
  Bus Selector : BusSelector  OutputSignals=d_ap1,d_ap2,d_ap3,d_ap4
  IGBT/Diode{,1..7} (8 alike) : spsIGBTDiodeLib/IGBT//Diode  Ron=1e-5  Rs=1e5  Cs=inf  Measurements=off
  Logical Operator{,1..3} (4 alike) : Logic  Operator=NOT  AllPortsSameDT=off  OutDataTypeStr=boolean
  Scope : Subsystem  LoadFcn=plecs('sl', 300);  InitFcn=plecs('sl', 314);  StartFcn=plecs('sl', 308);  StopFcn=plecs('sl', 309);  mask{Settings=<binary blob, 236 chars, not shown>}
      mask init:
      | plecs('sl', 315);
      settings: CopyFcn=plecs('sl', 303);  DeleteFcn=plecs('sl', 305);  UndoDeleteFcn=plecs('sl', 306);  PreSaveFcn=plecs('sl', 311);  NameChangeFcn=plecs('sl', 310);  DestroyFcn=plecs('sl', 307);  OpenFcn=plecs('sl', 302);  ErrorFcn=plerrorfcn
      mask Display: plot([0.1 0.9 0.9 0.1 0.1], [0.9 0.9 0.5 0.5 0.9])
  Scope1 : Subsystem  LoadFcn=plecs('sl', 300);  InitFcn=plecs('sl', 314);  StartFcn=plecs('sl', 308);  StopFcn=plecs('sl', 309);  mask{Settings=<binary blob, 236 chars, not shown>}
      mask init:
      | plecs('sl', 315);
      settings: CopyFcn=plecs('sl', 303);  DeleteFcn=plecs('sl', 305);  UndoDeleteFcn=plecs('sl', 306);  PreSaveFcn=plecs('sl', 311);  NameChangeFcn=plecs('sl', 310);  DestroyFcn=plecs('sl', 307);  OpenFcn=plecs('sl', 302);  ErrorFcn=plerrorfcn
      mask Display: plot([0.1 0.9 0.9 0.1 0.1], [0.9 0.9 0.5 0.5 0.9])
  Scope2 : Subsystem  LoadFcn=plecs('sl', 300);  InitFcn=plecs('sl', 314);  StartFcn=plecs('sl', 308);  StopFcn=plecs('sl', 309);  mask{Settings=<binary blob, 236 chars, not shown>}
      mask init:
      | plecs('sl', 315);
      settings: CopyFcn=plecs('sl', 303);  DeleteFcn=plecs('sl', 305);  UndoDeleteFcn=plecs('sl', 306);  PreSaveFcn=plecs('sl', 311);  NameChangeFcn=plecs('sl', 310);  DestroyFcn=plecs('sl', 307);  OpenFcn=plecs('sl', 302);  ErrorFcn=plerrorfcn
      mask Display: plot([0.1 0.9 0.9 0.1 0.1], [0.9 0.9 0.5 0.5 0.9])
  Scope3 : Subsystem  LoadFcn=plecs('sl', 300);  InitFcn=plecs('sl', 314);  StartFcn=plecs('sl', 308);  StopFcn=plecs('sl', 309);  mask{Settings=<binary blob, 236 chars, not shown>}
      mask init:
      | plecs('sl', 315);
      settings: CopyFcn=plecs('sl', 303);  DeleteFcn=plecs('sl', 305);  UndoDeleteFcn=plecs('sl', 306);  PreSaveFcn=plecs('sl', 311);  NameChangeFcn=plecs('sl', 310);  DestroyFcn=plecs('sl', 307);  OpenFcn=plecs('sl', 302);  ErrorFcn=plerrorfcn
      mask Display: plot([0.1 0.9 0.9 0.1 0.1], [0.9 0.9 0.5 0.5 0.9])
  Series RLC Branch{,1..3} (4 alike) : spsSeriesRLCBranchLib/Series RLC Branch  LConnTagsString=__new0  RConnTagsString=__new0  BranchType=C  Resistance=1  Inductance=1e-3  SetiL0=off  InitialCurrent=0  Capacitance=C_sm  Setx0=on  InitialVoltage=V0c  Measurements=None
  Voltage Measurement{,1..4} (5 alike) : spsVoltageMeasurementLib/Voltage Measurement  PhasorSimulation=off  OutputType=Complex  PSBequivalent=0
  + : PMIOPort  Side=Left
  - : PMIOPort  Port=2  Side=Right
  Vc_xy : Outport
  V_xy : Outport  Port=2
  wires:
  Voltage Measurement/1 -> Bus Creator/1  "Vc_ap1"
  Voltage Measurement1/1 -> Bus Creator/2  "Vc_ap2"
  Voltage Measurement2/1 -> Bus Creator/3  "Vc_ap3"
  Voltage Measurement3/1 -> Bus Creator/4  "Vc_ap4"
  Bus Creator/1 -> Vc_xy/1
  Logical Operator3/1 -> IGBT/Diode7/1
  Logical Operator2/1 -> IGBT/Diode5/1
  Logical Operator1/1 -> IGBT/Diode3/1
  Logical Operator/1 -> IGBT/Diode1/1
  Bus Selector/1 -> Scope/1(1), IGBT/Diode/1, Logical Operator/1  "<d_ap1>"
  Bus Selector/2 -> Scope1/1(1), Logical Operator1/1, IGBT/Diode2/1  "<d_ap2>"
  Bus Selector/3 -> Scope2/1(1), Logical Operator2/1, IGBT/Diode4/1  "<d_ap3>"
  Bus Selector/4 -> Scope3/1(1), Logical Operator3/1, IGBT/Diode6/1  "<d_ap4>"
  Voltage Measurement4/1 -> V_xy/1
  S_xy/1 -> Bus Selector/1
  connections:
  IGBT/Diode/RConn1 -- Voltage Measurement4/LConn1 -- +/RConn1 -- IGBT/Diode1/LConn1
  Series RLC Branch2/RConn1 -- Voltage Measurement2/LConn2 -- IGBT/Diode7/LConn1 -- IGBT/Diode6/RConn1 -- IGBT/Diode5/RConn1
  Series RLC Branch3/RConn1 -- Voltage Measurement3/LConn2 -- Voltage Measurement4/LConn2 -- -/RConn1 -- IGBT/Diode7/RConn1
  Series RLC Branch3/LConn1 -- Voltage Measurement3/LConn1 -- IGBT/Diode6/LConn1
  Series RLC Branch/LConn1 -- Voltage Measurement/LConn1 -- IGBT/Diode/LConn1
  Series RLC Branch1/RConn1 -- Voltage Measurement1/LConn2 -- IGBT/Diode5/LConn1 -- IGBT/Diode4/RConn1 -- IGBT/Diode3/RConn1
  Series RLC Branch/RConn1 -- Voltage Measurement/LConn2 -- IGBT/Diode1/RConn1 -- IGBT/Diode2/RConn1 -- IGBT/Diode3/LConn1
  Series RLC Branch2/LConn1 -- Voltage Measurement2/LConn1 -- IGBT/Diode4/LConn1
  Series RLC Branch1/LConn1 -- Voltage Measurement1/LConn1 -- IGBT/Diode2/LConn1

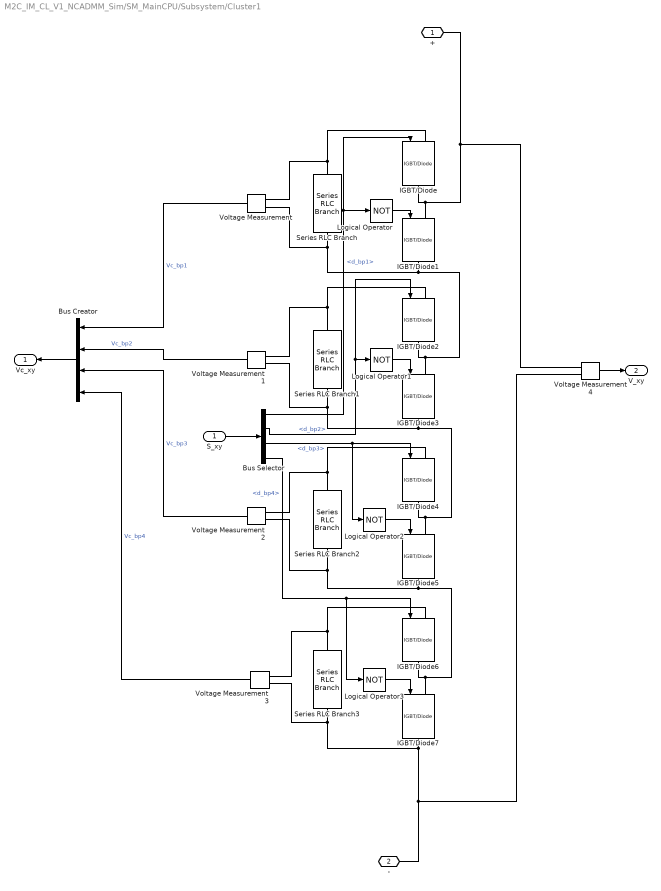
== system M2C_IM_CL_V1_NCADMM_Sim/SM_MainCPU/Subsystem/Cluster1 ==
  S_xy : Inport
  Bus Creator : BusCreator  Inputs=4
  Bus Selector : BusSelector  OutputSignals=d_bp1,d_bp2,d_bp3,d_bp4
  IGBT/Diode{,1..7} (8 alike) : spsIGBTDiodeLib/IGBT//Diode  Ron=1e-5  Rs=1e5  Cs=inf  Measurements=off
  Logical Operator{,1..3} (4 alike) : Logic  Operator=NOT  AllPortsSameDT=off  OutDataTypeStr=boolean
  Series RLC Branch{,1..3} (4 alike) : spsSeriesRLCBranchLib/Series RLC Branch  LConnTagsString=__new0  RConnTagsString=__new0  BranchType=C  Resistance=1  Inductance=1e-3  SetiL0=off  InitialCurrent=0  Capacitance=C_sm  Setx0=on  InitialVoltage=V0c  Measurements=None
  Voltage Measurement{,1..4} (5 alike) : spsVoltageMeasurementLib/Voltage Measurement  PhasorSimulation=off  OutputType=Complex  PSBequivalent=0
  + : PMIOPort  Side=Left
  - : PMIOPort  Port=2  Side=Right
  Vc_xy : Outport
  V_xy : Outport  Port=2
  wires:
  Bus Selector/4 -> IGBT/Diode6/1, Logical Operator3/1  "<d_bp4>"
  Bus Selector/3 -> IGBT/Diode4/1, Logical Operator2/1  "<d_bp3>"
  Bus Selector/2 -> IGBT/Diode2/1, Logical Operator1/1  "<d_bp2>"
  Bus Selector/1 -> Logical Operator/1, IGBT/Diode/1  "<d_bp1>"
  S_xy/1 -> Bus Selector/1
  Logical Operator/1 -> IGBT/Diode1/1
  Logical Operator1/1 -> IGBT/Diode3/1
  Logical Operator2/1 -> IGBT/Diode5/1
  Logical Operator3/1 -> IGBT/Diode7/1
  Bus Creator/1 -> Vc_xy/1
  Voltage Measurement3/1 -> Bus Creator/4  "Vc_bp4"
  Voltage Measurement2/1 -> Bus Creator/3  "Vc_bp3"
  Voltage Measurement1/1 -> Bus Creator/2  "Vc_bp2"
  Voltage Measurement/1 -> Bus Creator/1  "Vc_bp1"
  Voltage Measurement4/1 -> V_xy/1
  connections:
  Voltage Measurement1/LConn1 -- Series RLC Branch1/LConn1 -- IGBT/Diode2/LConn1
  Voltage Measurement2/LConn1 -- Series RLC Branch2/LConn1 -- IGBT/Diode4/LConn1
  Voltage Measurement/LConn2 -- Series RLC Branch/RConn1 -- IGBT/Diode3/LConn1 -- IGBT/Diode2/RConn1 -- IGBT/Diode1/RConn1
  Voltage Measurement1/LConn2 -- Series RLC Branch1/RConn1 -- IGBT/Diode3/RConn1 -- IGBT/Diode4/RConn1 -- IGBT/Diode5/LConn1
  Voltage Measurement/LConn1 -- Series RLC Branch/LConn1 -- IGBT/Diode/LConn1
  Voltage Measurement3/LConn1 -- Series RLC Branch3/LConn1 -- IGBT/Diode6/LConn1
  Voltage Measurement3/LConn2 -- Series RLC Branch3/RConn1 -- IGBT/Diode7/RConn1 -- Voltage Measurement4/LConn2 -- -/RConn1
  Voltage Measurement2/LConn2 -- Series RLC Branch2/RConn1 -- IGBT/Diode5/RConn1 -- IGBT/Diode6/RConn1 -- IGBT/Diode7/LConn1
  IGBT/Diode/RConn1 -- IGBT/Diode1/LConn1 -- Voltage Measurement4/LConn1 -- +/RConn1

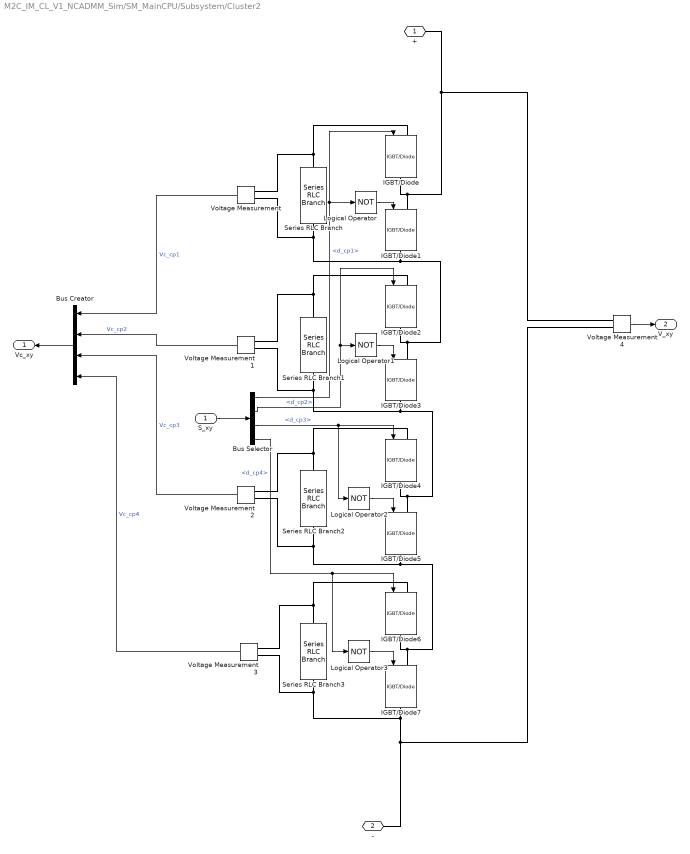
== system M2C_IM_CL_V1_NCADMM_Sim/SM_MainCPU/Subsystem/Cluster2 ==
  S_xy : Inport
  Bus Creator : BusCreator  Inputs=4
  Bus Selector : BusSelector  OutputSignals=d_cp1,d_cp2,d_cp3,d_cp4
  IGBT/Diode{,1..7} (8 alike) : spsIGBTDiodeLib/IGBT//Diode  Ron=1e-5  Rs=1e5  Cs=inf  Measurements=off
  Logical Operator{,1..3} (4 alike) : Logic  Operator=NOT  AllPortsSameDT=off  OutDataTypeStr=boolean
  Series RLC Branch{,1..3} (4 alike) : spsSeriesRLCBranchLib/Series RLC Branch  LConnTagsString=__new0  RConnTagsString=__new0  BranchType=C  Resistance=1  Inductance=1e-3  SetiL0=off  InitialCurrent=0  Capacitance=C_sm  Setx0=on  InitialVoltage=V0c  Measurements=None
  Voltage Measurement{,1..4} (5 alike) : spsVoltageMeasurementLib/Voltage Measurement  PhasorSimulation=off  OutputType=Complex  PSBequivalent=0
  + : PMIOPort  Side=Left
  - : PMIOPort  Port=2  Side=Right
  Vc_xy : Outport
  V_xy : Outport  Port=2
  wires:
  Voltage Measurement/1 -> Bus Creator/1  "Vc_cp1"
  Voltage Measurement1/1 -> Bus Creator/2  "Vc_cp2"
  Voltage Measurement2/1 -> Bus Creator/3  "Vc_cp3"
  Voltage Measurement3/1 -> Bus Creator/4  "Vc_cp4"
  Bus Creator/1 -> Vc_xy/1
  Logical Operator3/1 -> IGBT/Diode7/1
  Logical Operator2/1 -> IGBT/Diode5/1
  Logical Operator1/1 -> IGBT/Diode3/1
  Logical Operator/1 -> IGBT/Diode1/1
  S_xy/1 -> Bus Selector/1
  Bus Selector/1 -> IGBT/Diode/1, Logical Operator/1  "<d_cp1>"
  Bus Selector/2 -> Logical Operator1/1, IGBT/Diode2/1  "<d_cp2>"
  Bus Selector/3 -> Logical Operator2/1, IGBT/Diode4/1  "<d_cp3>"
  Bus Selector/4 -> Logical Operator3/1, IGBT/Diode6/1  "<d_cp4>"
  Voltage Measurement4/1 -> V_xy/1
  connections:
  IGBT/Diode1/LConn1 -- IGBT/Diode/RConn1 -- Voltage Measurement4/LConn1 -- +/RConn1
  IGBT/Diode7/LConn1 -- IGBT/Diode6/RConn1 -- IGBT/Diode5/RConn1 -- Series RLC Branch2/RConn1 -- Voltage Measurement2/LConn2
  IGBT/Diode7/RConn1 -- Series RLC Branch3/RConn1 -- Voltage Measurement3/LConn2 -- Voltage Measurement4/LConn2 -- -/RConn1
  IGBT/Diode6/LConn1 -- Series RLC Branch3/LConn1 -- Voltage Measurement3/LConn1
  IGBT/Diode/LConn1 -- Series RLC Branch/LConn1 -- Voltage Measurement/LConn1
  IGBT/Diode5/LConn1 -- IGBT/Diode4/RConn1 -- IGBT/Diode3/RConn1 -- Series RLC Branch1/RConn1 -- Voltage Measurement1/LConn2
  IGBT/Diode1/RConn1 -- IGBT/Diode2/RConn1 -- IGBT/Diode3/LConn1 -- Series RLC Branch/RConn1 -- Voltage Measurement/LConn2
  IGBT/Diode4/LConn1 -- Series RLC Branch2/LConn1 -- Voltage Measurement2/LConn1
  IGBT/Diode2/LConn1 -- Series RLC Branch1/LConn1 -- Voltage Measurement1/LConn1

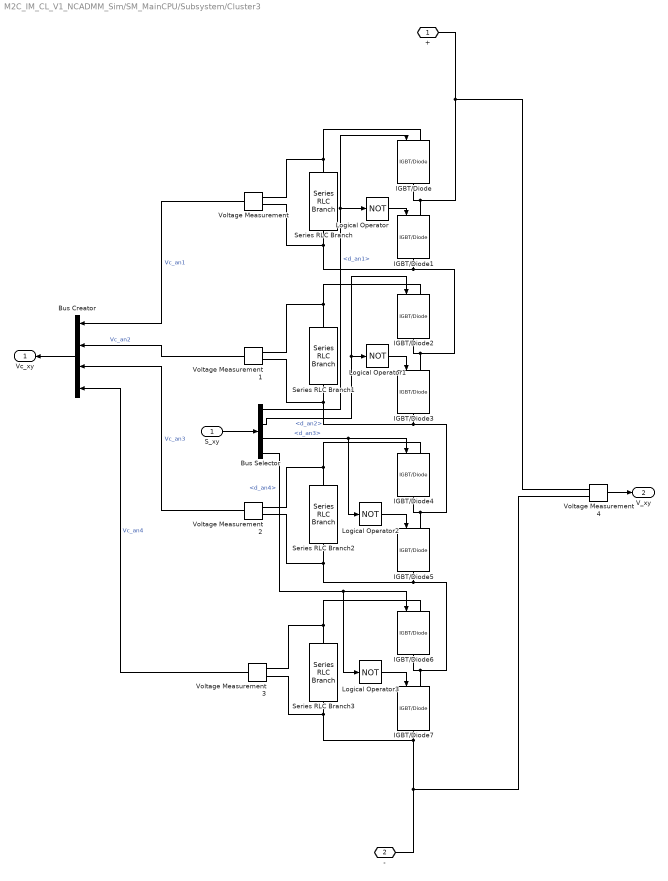
== system M2C_IM_CL_V1_NCADMM_Sim/SM_MainCPU/Subsystem/Cluster3 ==
  S_xy : Inport
  Bus Creator : BusCreator  Inputs=4
  Bus Selector : BusSelector  OutputSignals=d_an1,d_an2,d_an3,d_an4
  IGBT/Diode{,1..7} (8 alike) : spsIGBTDiodeLib/IGBT//Diode  Ron=1e-5  Rs=1e5  Cs=inf  Measurements=off
  Logical Operator{,1..3} (4 alike) : Logic  Operator=NOT  AllPortsSameDT=off  OutDataTypeStr=boolean
  Series RLC Branch{,1..3} (4 alike) : spsSeriesRLCBranchLib/Series RLC Branch  LConnTagsString=__new0  RConnTagsString=__new0  BranchType=C  Resistance=1  Inductance=1e-3  SetiL0=off  InitialCurrent=0  Capacitance=C_sm  Setx0=on  InitialVoltage=V0c  Measurements=None
  Voltage Measurement{,1..4} (5 alike) : spsVoltageMeasurementLib/Voltage Measurement  PhasorSimulation=off  OutputType=Complex  PSBequivalent=0
  + : PMIOPort  Side=Left
  - : PMIOPort  Port=2  Side=Right
  Vc_xy : Outport
  V_xy : Outport  Port=2
  wires:
  Bus Selector/4 -> IGBT/Diode6/1, Logical Operator3/1  "<d_an4>"
  Bus Selector/3 -> IGBT/Diode4/1, Logical Operator2/1  "<d_an3>"
  Bus Selector/2 -> IGBT/Diode2/1, Logical Operator1/1  "<d_an2>"
  Bus Selector/1 -> Logical Operator/1, IGBT/Diode/1  "<d_an1>"
  S_xy/1 -> Bus Selector/1
  Logical Operator/1 -> IGBT/Diode1/1
  Logical Operator1/1 -> IGBT/Diode3/1
  Logical Operator2/1 -> IGBT/Diode5/1
  Logical Operator3/1 -> IGBT/Diode7/1
  Bus Creator/1 -> Vc_xy/1
  Voltage Measurement3/1 -> Bus Creator/4  "Vc_an4"
  Voltage Measurement2/1 -> Bus Creator/3  "Vc_an3"
  Voltage Measurement1/1 -> Bus Creator/2  "Vc_an2"
  Voltage Measurement/1 -> Bus Creator/1  "Vc_an1"
  Voltage Measurement4/1 -> V_xy/1
  connections:
  Voltage Measurement1/LConn1 -- Series RLC Branch1/LConn1 -- IGBT/Diode2/LConn1
  Voltage Measurement2/LConn1 -- Series RLC Branch2/LConn1 -- IGBT/Diode4/LConn1
  Voltage Measurement/LConn2 -- Series RLC Branch/RConn1 -- IGBT/Diode3/LConn1 -- IGBT/Diode2/RConn1 -- IGBT/Diode1/RConn1
  Voltage Measurement1/LConn2 -- Series RLC Branch1/RConn1 -- IGBT/Diode3/RConn1 -- IGBT/Diode4/RConn1 -- IGBT/Diode5/LConn1
  Voltage Measurement/LConn1 -- Series RLC Branch/LConn1 -- IGBT/Diode/LConn1
  Voltage Measurement3/LConn1 -- Series RLC Branch3/LConn1 -- IGBT/Diode6/LConn1
  Voltage Measurement3/LConn2 -- Series RLC Branch3/RConn1 -- IGBT/Diode7/RConn1 -- Voltage Measurement4/LConn1 -- -/RConn1
  Voltage Measurement2/LConn2 -- Series RLC Branch2/RConn1 -- IGBT/Diode5/RConn1 -- IGBT/Diode6/RConn1 -- IGBT/Diode7/LConn1
  IGBT/Diode/RConn1 -- IGBT/Diode1/LConn1 -- Voltage Measurement4/LConn2 -- +/RConn1

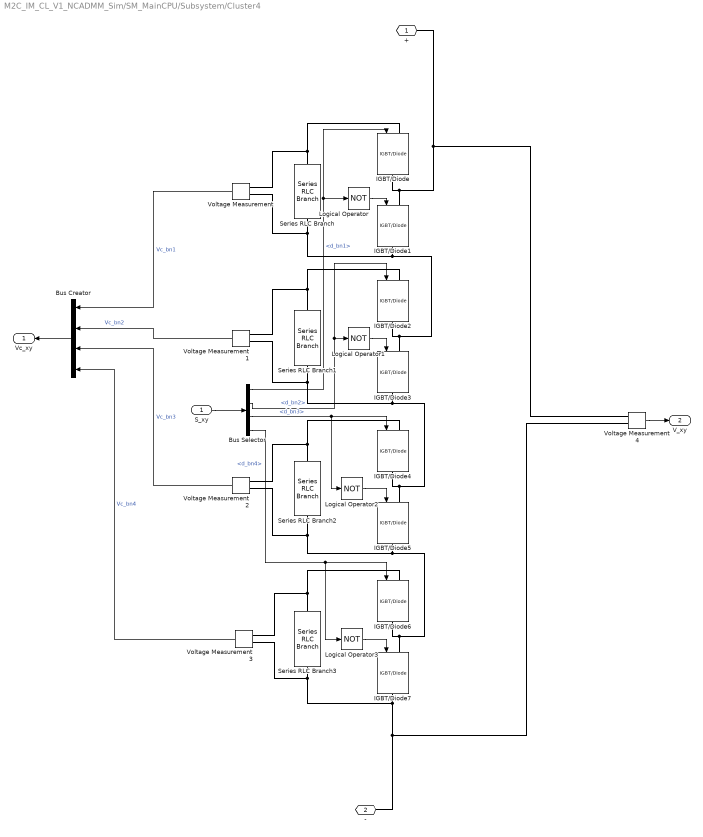
== system M2C_IM_CL_V1_NCADMM_Sim/SM_MainCPU/Subsystem/Cluster4 ==
  S_xy : Inport
  Bus Creator : BusCreator  Inputs=4
  Bus Selector : BusSelector  OutputSignals=d_bn1,d_bn2,d_bn3,d_bn4
  IGBT/Diode{,1..7} (8 alike) : spsIGBTDiodeLib/IGBT//Diode  Ron=1e-5  Rs=1e5  Cs=inf  Measurements=off
  Logical Operator{,1..3} (4 alike) : Logic  Operator=NOT  AllPortsSameDT=off  OutDataTypeStr=boolean
  Series RLC Branch{,1..3} (4 alike) : spsSeriesRLCBranchLib/Series RLC Branch  LConnTagsString=__new0  RConnTagsString=__new0  BranchType=C  Resistance=1  Inductance=1e-3  SetiL0=off  InitialCurrent=0  Capacitance=C_sm  Setx0=on  InitialVoltage=V0c  Measurements=None
  Voltage Measurement{,1..4} (5 alike) : spsVoltageMeasurementLib/Voltage Measurement  PhasorSimulation=off  OutputType=Complex  PSBequivalent=0
  + : PMIOPort  Side=Left
  - : PMIOPort  Port=2  Side=Right
  Vc_xy : Outport
  V_xy : Outport  Port=2
  wires:
  Voltage Measurement/1 -> Bus Creator/1  "Vc_bn1"
  Voltage Measurement1/1 -> Bus Creator/2  "Vc_bn2"
  Voltage Measurement2/1 -> Bus Creator/3  "Vc_bn3"
  Voltage Measurement3/1 -> Bus Creator/4  "Vc_bn4"
  Bus Creator/1 -> Vc_xy/1
  Logical Operator3/1 -> IGBT/Diode7/1
  Logical Operator2/1 -> IGBT/Diode5/1
  Logical Operator1/1 -> IGBT/Diode3/1
  Logical Operator/1 -> IGBT/Diode1/1
  S_xy/1 -> Bus Selector/1
  Bus Selector/1 -> IGBT/Diode/1, Logical Operator/1  "<d_bn1>"
  Bus Selector/2 -> Logical Operator1/1, IGBT/Diode2/1  "<d_bn2>"
  Bus Selector/3 -> Logical Operator2/1, IGBT/Diode4/1  "<d_bn3>"
  Bus Selector/4 -> Logical Operator3/1, IGBT/Diode6/1  "<d_bn4>"
  Voltage Measurement4/1 -> V_xy/1
  connections:
  IGBT/Diode1/LConn1 -- IGBT/Diode/RConn1 -- Voltage Measurement4/LConn2 -- +/RConn1
  IGBT/Diode7/LConn1 -- IGBT/Diode6/RConn1 -- IGBT/Diode5/RConn1 -- Series RLC Branch2/RConn1 -- Voltage Measurement2/LConn2
  IGBT/Diode7/RConn1 -- Series RLC Branch3/RConn1 -- Voltage Measurement3/LConn2 -- Voltage Measurement4/LConn1 -- -/RConn1
  IGBT/Diode6/LConn1 -- Series RLC Branch3/LConn1 -- Voltage Measurement3/LConn1
  IGBT/Diode/LConn1 -- Series RLC Branch/LConn1 -- Voltage Measurement/LConn1
  IGBT/Diode5/LConn1 -- IGBT/Diode4/RConn1 -- IGBT/Diode3/RConn1 -- Series RLC Branch1/RConn1 -- Voltage Measurement1/LConn2
  IGBT/Diode1/RConn1 -- IGBT/Diode2/RConn1 -- IGBT/Diode3/LConn1 -- Series RLC Branch/RConn1 -- Voltage Measurement/LConn2
  IGBT/Diode4/LConn1 -- Series RLC Branch2/LConn1 -- Voltage Measurement2/LConn1
  IGBT/Diode2/LConn1 -- Series RLC Branch1/LConn1 -- Voltage Measurement1/LConn1
